simulink model "untitled"  (R2019b)
settings: Solver=VariableStepAuto  StartTime=0.0  StopTime=10.0  RelTol=1e-3
settings Model: Creator=Chris  LastModifiedBy=Chris

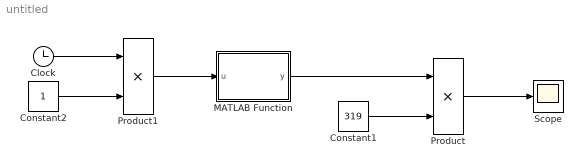
== system untitled ==
  Clock : Clock
  Constant1 : Constant  Value=319
  Constant2 : Constant
  MATLAB Function : MATLAB Function  TreatAsAtomicUnit=on
  Product : Product
  Product1 : Product
  Scope : Scope
  wires:
  MATLAB Function/1(y) -> Product/1
  Constant1/1 -> Product/2
  Product/1 -> Scope/1
  Clock/1 -> Product1/1
  Constant2/1 -> Product1/2
  Product1/1 -> MATLAB Function/1(u)

== matlab function untitled/MATLAB Function ==
  data: u input; y output
function y = fcn(u)
    persistent time
    time = 5;
    if(u==1)
        timer = tic;
        time = time - toc(timer);
        y = 1;
    else
        y = 0;
    end
end
